simulink model "Control_con_realimentacion_estado_usando_observador"  (R2015a)
settings: Solver=ode5  StartTime=0.0  StopTime=18  FixedStep=0.001  RelTol=1e-3
values from neighbouring files (symbols this model uses):
  A = [0,0,1,0;0,0,0,1;0,Ks/Ms,-Be*(Ms+Mc)/(Ms*Mc),0;0,-Ks/Ms,Be/Ms,0]    [Par_sistema_edif_amd.m]
  B = [0;0;K*(Ms+Mc)/(Mc*Ms);-K/Ms]    [Par_sistema_edif_amd.m]
  Be = (Kg^2*Kt^2)/(rmp^2*Rm)    (= 7.72356398165)    [Par_sistema_edif_amd.m]
  C = [1,0,0,0;0,-Ks/Ms,Be/Ms,0]    [Par_sistema_edif_amd.m]
  D = [0;-K/Ms]    [Par_sistema_edif_amd.m]
  K = Kg*Kt/(rmp*Rm)    (= 1.72354330709)    [Par_sistema_edif_amd.m]
  Kc = acker(A,B,J)    [Par_sistema_edif_amd.m]
  Ko = place(A',C',L)'    [Par_sistema_edif_amd.m]
  Ks = 500.8824    [Par_sistema_edif_amd.m]
  Mc = 0.65    [Par_sistema_edif_amd.m]
  Ms = 1.6    [Par_sistema_edif_amd.m]
settings Model: ExtModeTrigDuration=10000  Creator=Usuario  LastModifiedBy=Usuario
settings SolverCC: PositivePriorityOrder=on
settings RTWCC: SystemTargetFile=quarc_win64.tlc  TemplateMakefile=quarc_default_tmf  Description=QUARC Win64 Target
settings STFCustomTargetCC: TargetLibSuffix=.lib  TargetPreCompLibLocation=C:\PROGRA~3\QUARC\lib\2015a\win64\release  GenerateSampleERTMain=off  ConcurrentExecutionCompliant=on  GeneratePreprocessorConditionals=Disable all  ERTCustomFileBanners=off  SupportNonInlinedSFcns=on  SupportVariableSizeSignals=off  MATLABClassNameForMDSCustomization=Simulink.SoftwareTarget.GRTCustomization  GRTInterface=on  SystemTargetFile=quarc_win64.tlc
settings GRTTargetCC: TargetPreCompLibLocation=C:\PROGRA~3\QUARC\lib\2015a\win64\release  ParMdlRefBuildCompliant=off  CompOptLevelCompliant=off  CombineOutputUpdateFcns=off  MatFileLogging=off  CPPClassGenCompliant=off  GRTInterface=on  ExtMode=on  ExtModeMexFile=quarc_comm

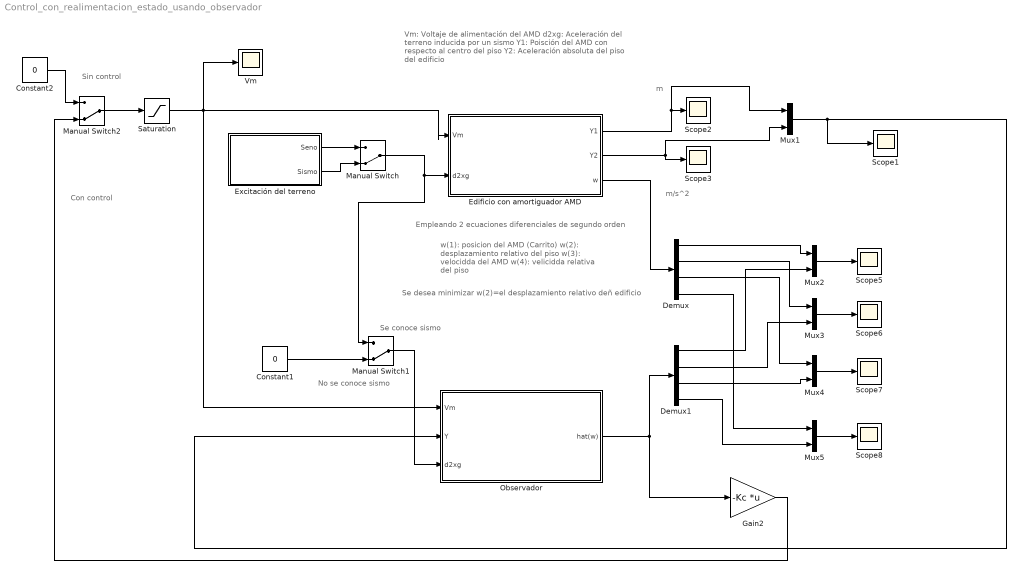
== system Control_con_realimentacion_estado_usando_observador ==
  note: w(1): posicion del AMD (Carrito)
      | w(2): desplazamiento relativo del piso
      | w(3): velocidda del AMD
      | w(4): velicidda relativa del piso
  note: Se desea minimizar w(2)=el desplazamiento relativo deñ edificio
  note: Sin control
  note: Con control
  note: No se conoce sismo
  note: Se conoce sismo
  note: m/s^2
  note: m
  note: Empleando 2 ecuaciones diferenciales de segundo orden
  note: Vm: Voltaje de alimentación del AMD
      | d2xg: Aceleración del terreno inducida por un sismo
      | Y1: Poisción del AMD con respecto al centro del piso
      | Y2: Aceleración absoluta del piso del edificio
  Constant1 : Constant  Value=0
  Constant2 : Constant  Value=0
  Demux : Demux
  Demux1 : Demux
  Edificio con amortiguador AMD : Subsystem
  Excitación del terreno : Subsystem
  Gain2 : Gain  Gain=-Kc  Multiplication=Matrix(K*u)
  Manual Switch : ManualSwitch  CurrentSetting=0
  Manual Switch1 : ManualSwitch  CurrentSetting=0
  Manual Switch2 : ManualSwitch  CurrentSetting=0
  Mux{1..5} (5 alike) : Mux  Inputs=2
  Observador : Subsystem
  Saturation : Saturate  UpperLimit=10  LowerLimit=-10
  Scope{1..3,5..8} (7 alike) : Scope
      Scope2 settings: SaveName=ScopeData2
      Scope3 settings: SaveName=ScopeData3
      Scope5 settings: SaveName=ScopeData10
      Scope6 settings: SaveName=ScopeData11
      Scope7 settings: SaveName=ScopeData12
      Scope8 settings: SaveName=ScopeData13
  Vm : Scope
  wires:
  Edificio con amortiguador AMD/2(Y2) -> Scope3/1, Mux1/2
  Saturation/1 -> Observador/1(Vm), Vm/1, Edificio con amortiguador AMD/1(Vm)
  Edificio con amortiguador AMD/1(Y1) -> Mux1/1, Scope2/1
  Mux1/1 -> Observador/2(Y), Scope1/1
  Excitación del terreno/1(Seno) -> Manual Switch/1
  Excitación del terreno/2(Sismo) -> Manual Switch/2
  Manual Switch/1 -> Manual Switch1/1, Edificio con amortiguador AMD/2(d2xg)
  Gain2/1 -> Manual Switch2/2
  Observador/1(hat(w)) -> Demux1/1, Gain2/1
  Edificio con amortiguador AMD/3(w) -> Demux/1
  Demux/1 -> Mux2/1
  Demux1/1 -> Mux2/2
  Demux/2 -> Mux3/1
  Demux1/2 -> Mux3/2
  Demux/3 -> Mux4/1
  Demux1/3 -> Mux4/2
  Demux/4 -> Mux5/1
  Demux1/4 -> Mux5/2
  Mux2/1 -> Scope5/1
  Mux3/1 -> Scope6/1
  Mux4/1 -> Scope7/1
  Mux5/1 -> Scope8/1
  Manual Switch1/1 -> Observador/3(d2xg)
  Constant1/1 -> Manual Switch1/2
  Manual Switch2/1 -> Saturation/1
  Constant2/1 -> Manual Switch2/1

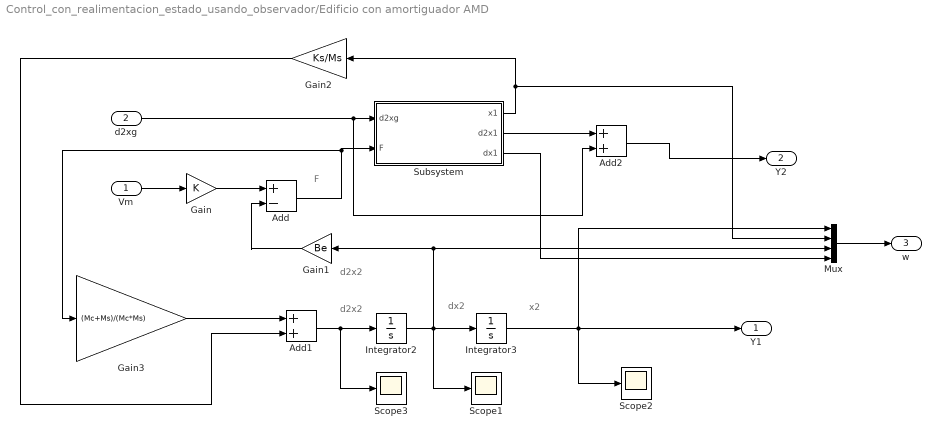
== system Control_con_realimentacion_estado_usando_observador/Edificio con amortiguador AMD ==
  note: d2x2
  note: F
  note: x2
  note: dx2
  note: d2x2
  Vm : Inport
  d2xg : Inport  Port=2
  Add : Sum  Inputs=+-
  Add1 : Sum
  Add2 : Sum
  Gain : Gain  Gain=K
  Gain1 : Gain  Gain=Be
  Gain2 : Gain  Gain=Ks/Ms
  Gain3 : Gain  Gain=(Mc+Ms)/(Mc*Ms)
  Integrator2 : Integrator
  Integrator3 : Integrator
  Mux : Mux
  Scope1 : Scope
      settings: SaveName=ScopeData8
  Scope2 : Scope
      settings: SaveName=ScopeData7
  Scope3 : Scope
      settings: SaveName=ScopeData9
  Subsystem : Subsystem
  Y1 : Outport
  Y2 : Outport  Port=2
  w : Outport  Port=3
  wires:
  Gain3/1 -> Add1/1
  Add1/1 -> Scope3/1, Integrator2/1
  Subsystem/2(d2x1) -> Add2/1
  Gain/1 -> Add/1
  Gain2/1 -> Add1/2
  d2xg/1 -> Subsystem/1(d2xg), Add2/2
  Add/1 -> Gain3/1, Subsystem/2(F)
  Vm/1 -> Gain/1
  Gain1/1 -> Add/2
  Integrator2/1 -> Mux/3, Gain1/1, Scope1/1, Integrator3/1
  Add2/1 -> Y2/1
  Integrator3/1 -> Mux/1, Scope2/1, Y1/1
  Subsystem/1(x1) -> Gain2/1, Mux/2
  Subsystem/3(dx1) -> Mux/4
  Mux/1 -> w/1

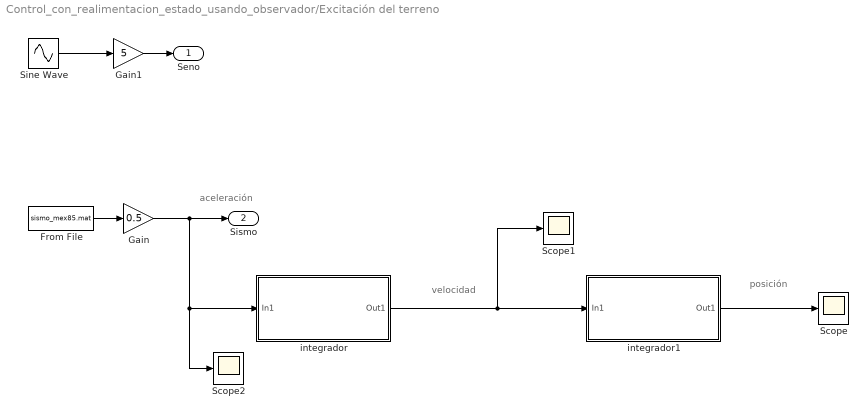
== system Control_con_realimentacion_estado_usando_observador/Excitación del terreno ==
  note: posición
  note: velocidad
  note: aceleración
  From File : FromFile  FileName=sismo_mex85.mat  SampleTime=0.001
  Gain : Gain  Gain=0.5
  Gain1 : Gain  Gain=5
  Scope : Scope
      settings: SaveName=ScopeData14
  Scope1 : Scope
      settings: SaveName=ScopeData15
  Scope2 : Scope
      settings: SaveName=ScopeData16
  Sine Wave : Sin  SampleTime=0
  integrador : Subsystem
  integrador1 : Subsystem
  Seno : Outport
  Sismo : Outport  Port=2
  wires:
  Gain/1 -> Scope2/1, integrador/1(In1), Sismo/1
  Sine Wave/1 -> Gain1/1
  From File/1 -> Gain/1
  integrador/1(Out1) -> Scope1/1, integrador1/1(In1)
  integrador1/1(Out1) -> Scope/1
  Gain1/1 -> Seno/1

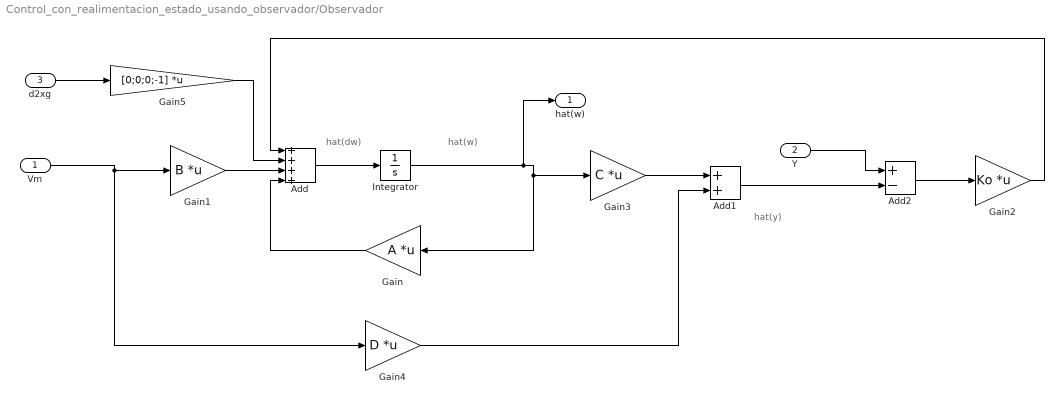
== system Control_con_realimentacion_estado_usando_observador/Observador ==
  note: hat(y)
  note: hat(w)
  note: hat(dw)
  Vm : Inport
  Y : Inport  Port=2
  d2xg : Inport  Port=3
  Add : Sum  Inputs=++++
  Add1 : Sum
  Add2 : Sum  Inputs=+-
  Gain : Gain  Gain=A  Multiplication=Matrix(K*u)
  Gain1 : Gain  Gain=B  Multiplication=Matrix(K*u)
  Gain2 : Gain  Gain=Ko  Multiplication=Matrix(K*u)
  Gain3 : Gain  Gain=C  Multiplication=Matrix(K*u)
  Gain4 : Gain  Gain=D  Multiplication=Matrix(K*u)
  Gain5 : Gain  Gain=[0;0;0;-1]  Multiplication=Matrix(K*u)
  Integrator : Integrator
  hat(w) : Outport
  wires:
  Integrator/1 -> hat(w)/1, Gain3/1, Gain/1
  Gain4/1 -> Add1/2
  Add/1 -> Integrator/1
  Gain3/1 -> Add1/1
  Vm/1 -> Gain4/1, Gain1/1
  Y/1 -> Add2/1
  Add1/1 -> Add2/2
  Add2/1 -> Gain2/1
  Gain2/1 -> Add/1
  Gain/1 -> Add/4
  Gain1/1 -> Add/3
  d2xg/1 -> Gain5/1
  Gain5/1 -> Add/2

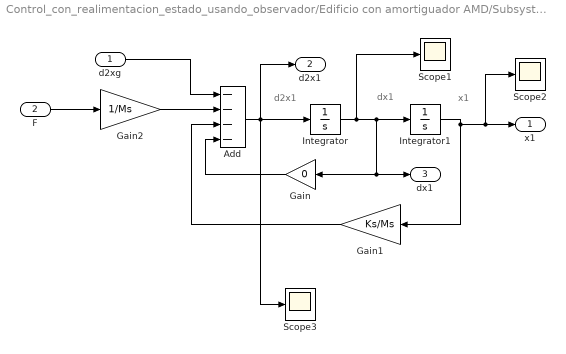
== system Control_con_realimentacion_estado_usando_observador/Edificio con amortiguador AMD/Subsystem ==
  note: x1
  note: dx1
  note: d2x1
  d2xg : Inport
  F : Inport  Port=2
  Add : Sum  Inputs=----
  Gain : Gain  Gain=0
  Gain1 : Gain  Gain=Ks/Ms
  Gain2 : Gain  Gain=1/Ms
  Integrator : Integrator
  Integrator1 : Integrator
  Scope1 : Scope
      settings: SaveName=ScopeData5
  Scope2 : Scope
      settings: SaveName=ScopeData4
  Scope3 : Scope
      settings: SaveName=ScopeData6
  x1 : Outport
  d2x1 : Outport  Port=2
  dx1 : Outport  Port=3
  wires:
  Add/1 -> d2x1/1, Scope3/1, Integrator/1
  Integrator/1 -> Scope1/1, dx1/1, Gain/1, Integrator1/1
  Integrator1/1 -> Scope2/1, x1/1, Gain1/1
  Gain1/1 -> Add/3
  Gain2/1 -> Add/2
  F/1 -> Gain2/1
  Gain/1 -> Add/4
  d2xg/1 -> Add/1

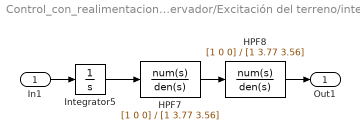
== system Control_con_realimentacion_estado_usando_observador/Excitación del terreno/integrador ==
  In1 : Inport
  HPF7 : TransferFcn  Numerator=[1 0 0]  Denominator=[1 3.77 3.56]
  HPF8 : TransferFcn  Numerator=[1 0 0]  Denominator=[1 3.77 3.56]
  Integrator5 : Integrator
  Out1 : Outport
  wires:
  HPF7/1 -> HPF8/1
  Integrator5/1 -> HPF7/1
  HPF8/1 -> Out1/1
  In1/1 -> Integrator5/1

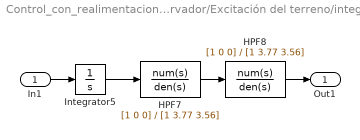
== system Control_con_realimentacion_estado_usando_observador/Excitación del terreno/integrador1 ==
  In1 : Inport
  HPF7 : TransferFcn  Numerator=[1 0 0]  Denominator=[1 3.77 3.56]
  HPF8 : TransferFcn  Numerator=[1 0 0]  Denominator=[1 3.77 3.56]
  Integrator5 : Integrator
  Out1 : Outport
  wires:
  HPF7/1 -> HPF8/1
  Integrator5/1 -> HPF7/1
  HPF8/1 -> Out1/1
  In1/1 -> Integrator5/1
